simulink model "j1s"  (R2023b)
settings: Solver=VariableStepAuto  StartTime=0.0  StopTime=20  RelTol=1e-3
settings Model: Creator=asus  LastModifiedBy=asus

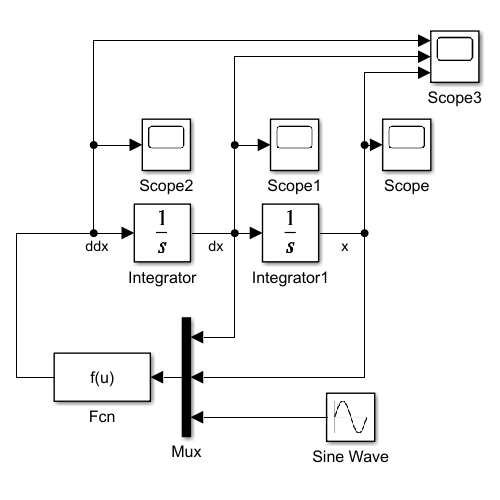
[thumbnail: Simulink's stored preview of the top-level diagram]
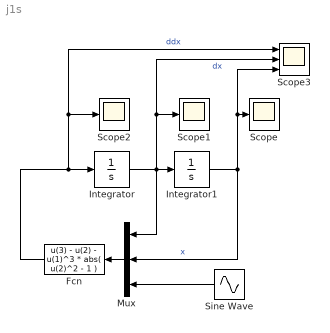
== system j1s ==
  Fcn : Fcn  Expr=u(3) - u(2) - u(1)^3 * abs( u(2)^2 - 1 )
  Integrator : Integrator  InitialCondition=1
  Integrator1 : Integrator  InitialCondition=1
  Mux : Mux  Inputs=3
  Scope : Scope
  Scope1 : Scope
  Scope2 : Scope
  Scope3 : Scope  NumInputPorts=3
  Sine Wave : Sin  Frequency=pi/2  SampleTime=0
  wires:
  Integrator/1 -> Scope3/2, Scope1/1, Mux/1, Integrator1/1  "dx"
  Integrator1/1 -> Scope3/3, Scope/1, Mux/2  "x"
  Fcn/1 -> Scope3/1, Scope2/1, Integrator/1  "ddx"
  Sine Wave/1 -> Mux/3
  Mux/1 -> Fcn/1
